simulink model "pemancar_bpsk"  (R2023a)
settings: Solver=FixedStepDiscrete  StartTime=0.0  StopTime=10.0  RelTol=1e-3
libraries: commrandsrc3 x1, hdlsllib x1, dspsrcs4 x1
settings Model: DataTypeOverride=Off  Creator=acer  LastModifiedBy=acer
settings SolverCC: AutoInsertRateTranBlk=on
settings OptimizationCC: BlockReduction=off  ConditionallyExecuteInputs=off  DefaultParameterBehavior=Inlined  InheritOutputTypeSmallerThanSingle=on
settings DebuggingCC: AlgebraicLoopMsg=error  SingleTaskRateTransMsg=error
settings HardwareCC: ProdBitPerPointer=32  ProdBitPerSizeT=32  ProdBitPerPtrDiffT=32  ProdLargestAtomicFloat=None  ProdIntDivRoundTo=Undefined  ProdEndianess=Unspecified  ProdWordSize=32  ProdHWDeviceType=ASIC/FPGA->ASIC/FPGA  TargetBitPerPointer=64  TargetBitPerSizeT=64  TargetBitPerPtrDiffT=64  TargetLongLongMode=on  TargetIntDivRoundTo=Zero  TargetEndianess=LittleEndian  TargetWordSize=64  TargetHWDeviceType=Custom Processor->MATLAB Host Computer  ProdEqTarget=off
settings ModelReferenceCC: EnableRefExpFcnMdlSchedulingChecks=on

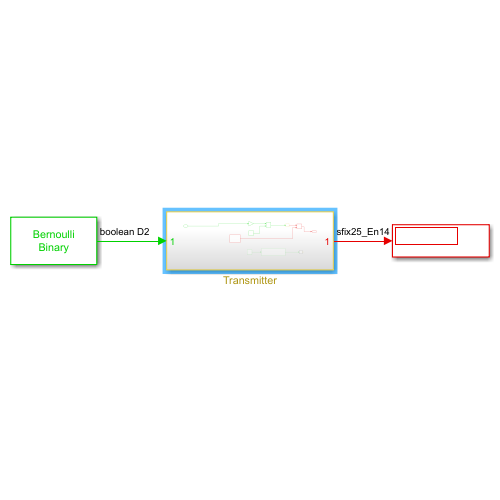
[thumbnail: Simulink's stored preview of the top-level diagram]
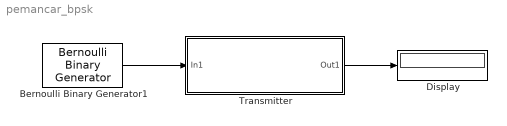
== system pemancar_bpsk ==
  Bernoulli Binary Generator1 : commrandsrc3/Bernoulli Binary Generator  ProbabilityOfZero=0.5  SeedSource=Parameter  Seed=32  SampleTime=1  SamplesPerFrame=1  OutputDataType=boolean  SimulateUsing=Interpreted execution
  Display : Display
  Transmitter : Subsystem
  wires:
  Bernoulli Binary Generator1/1 -> Transmitter/1(In1)
  Transmitter/1(Out1) -> Display/1

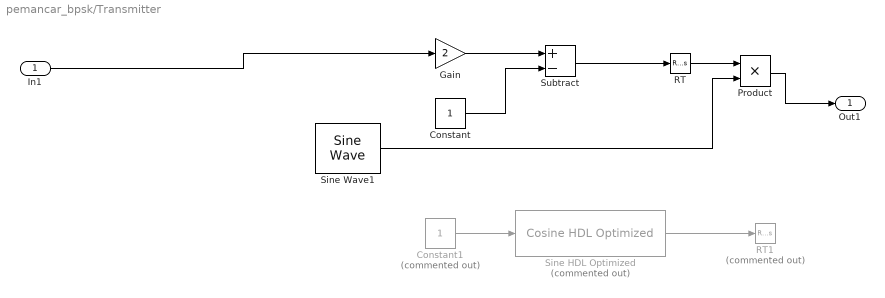
== system pemancar_bpsk/Transmitter ==
  In1 : Inport
  Constant : Constant  OutDataTypeStr=uint8  SampleTime=1
  Constant1 : Constant  Commented=on  OutDataTypeStr=uint8  SampleTime=1
  Gain : Gain  Gain=2
  Product : Product
  RT : RateTransition  OutPortSampleTime=0.001
  RT1 : RateTransition  Commented=on  OutPortSampleTime=0.001
  Sine HDL Optimized : hdlsllib/Lookup Tables/Cosine HDL Optimized  Commented=on  OutputFormula=sin(2*pi*u)  NumDataPoints=64  TableDataTypeStr=fixdt(0,16,15)  SimulateLUTROMDelay=off
      settings: LibrarySourceBlock=|
      | hdlsllib/Lookup
      | Tables/Sine
      | HDL Optimized
  Sine Wave1 : dspsrcs4/Sine Wave  Amplitude=1  Frequency=500  Phase=0.5*pi  SampleMode=Discrete  OutComplex=Real  CompMethod=Table lookup  TableSize=Speed  SampleTime=1/1000  SamplesPerFrame=1  ResetState=Restart at time zero  OutputFrames=off  dataType=Fixed-point  wordLen=16  udDataType=sfix(16)  fracBitsMode=Best precision  numFracBits=14  OutDataTypeStr=fixdt(1,16)  LastOutDataTypeStr=fixdt(1,16)
  Subtract : Sum  Inputs=+-
  Out1 : Outport
  wires:
  Constant/1 -> Subtract/2
  RT/1 -> Product/1
  Subtract/1 -> RT/1
  Gain/1 -> Subtract/1
  Product/1 -> Out1/1
  In1/1 -> Gain/1
  Constant1/1 -> Sine HDL Optimized/1
  Sine HDL Optimized/1 -> RT1/1
  Sine Wave1/1 -> Product/2
